simulink model "KITTDynamicsFinal"  (R2015b)
settings: Solver=FixedStepAuto  StartTime=0.0  StopTime=8  FixedStep=0.01  RelTol=1e-3
values from neighbouring files (symbols this model uses):
  b = 0.0015    [KITTParameters.m]
  c = 0.02    [KITTParameters.m]    (also in directionkeys.m = 0)
  m = 13    [KITTParameters.m]
undefined symbols (not defined in the file or in its folder): magnitude
settings Model: Creator=koenm  LastModifiedBy=koenm
settings DataIOCC: SaveFormat=StructureWithTime
settings DebuggingCC: AlgebraicLoopMsg=none

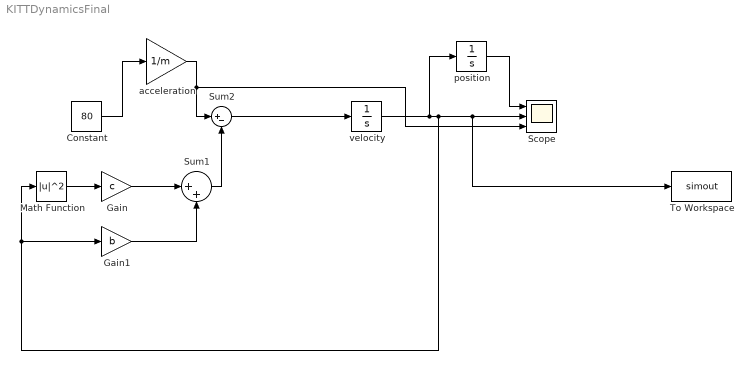
== system KITTDynamicsFinal ==
  Constant : Constant  Value=80
  Gain : Gain  Gain=c
  Gain1 : Gain  Gain=b
  Math Function : Math  Operator=magnitude^2  SaturateOnIntegerOverflow=on
  Scope : Scope  NumInputPorts=3
  Sum1 : Sum  Inputs=|++
  Sum2 : Sum  Inputs=|+-
  To Workspace : ToWorkspace  VariableName=simout  SaveFormat=Timeseries  SampleTime=-1
  acceleration : Gain  Gain=1/m
  position : Integrator
  velocity : Integrator  InitialCondition=1
  wires:
  Math Function/1 -> Gain/1
  Gain/1 -> Sum1/1
  Gain1/1 -> Sum1/2
  position/1 -> Scope/1
  Sum1/1 -> Sum2/2
  velocity/1 -> position/1, Gain1/1, Math Function/1, To Workspace/1, Scope/2
  Sum2/1 -> velocity/1
  Constant/1 -> acceleration/1
  acceleration/1 -> Scope/3, Sum2/1
